simulink model "pr733_DUC_modulation"  (R2018b)
settings: Solver=VariableStepAuto  StartTime=0.0  StopTime=8192/fs  RelTol=1e-3
PreLoadFcn:
  | fs=1e8;
  | pr731_DUC_setup;
  | fc=40e6;
undefined symbols (not defined in the file or in its folder): CFIR, CIC, designMultirateFIR, RRC
libraries: dspmlti4 x6, commrandsrc3 x1, commdigbbndpm3 x1
settings Model: Creator=Григорий Фокин  LastModifiedBy=Григорий Фокин
settings DataIOCC: SaveFormat=Array  SaveOutput=off  SignalLogging=off  SaveTime=off
settings DebuggingCC: AlgebraicLoopMsg=error
settings HardwareCC: ProdBitPerPointer=32  ProdBitPerSizeT=32  ProdBitPerPtrDiffT=32  ProdLargestAtomicFloat=None  ProdIntDivRoundTo=Undefined  ProdEndianess=Unspecified  ProdWordSize=32  ProdHWDeviceType=ASIC/FPGA->ASIC/FPGA  TargetBitPerPointer=64  TargetBitPerSizeT=64  TargetBitPerPtrDiffT=64  TargetLongLongMode=on  TargetIntDivRoundTo=Zero  TargetEndianess=LittleEndian  TargetWordSize=64  TargetHWDeviceType=Custom Processor->MATLAB Host Computer  ProdEqTarget=off

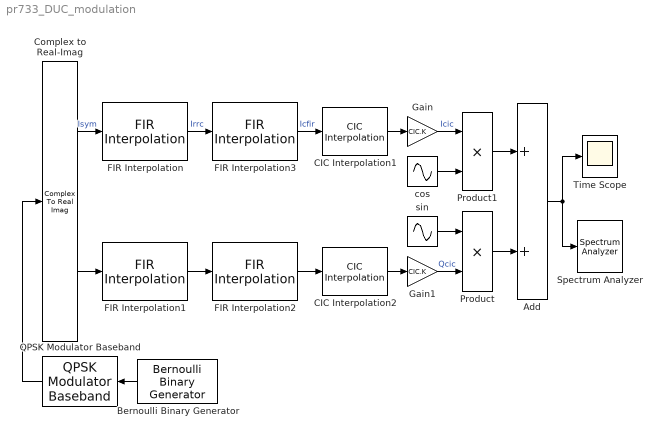
== system pr733_DUC_modulation ==
  Add : Sum
  Bernoulli Binary Generator : commrandsrc3/Bernoulli Binary Generator  ProbabilityOfZero=0.5  SeedSource=Auto  Seed=0  SampleTime=(0.5*CIC.R*RRC.Lfactor*CFIR.Lfactor)/fs  SamplesPerFrame=2  OutputDataType=boolean  SimulateUsing=Interpreted execution
  CIC Interpolation1 : dspmlti4/CIC Interpolation  filtFrom=Multirate object in workspace  filtobj=hCIC  ftype=Interpolator  R=2  M=1  N=2  filterInternals=Full precision  BPS=[16 16 16 16]  FLPS=0  outputWordLength=32  outputFracLength=0  launchFVT=off  framing=Allow multirate processing  OutputFrames=off
      settings: SourceProductName=DSP System Toolbox  SourceProductBaseCode=DS
  CIC Interpolation2 : dspmlti4/CIC Interpolation  filtFrom=Multirate object in workspace  filtobj=hCIC  ftype=Interpolator  R=2  M=1  N=2  filterInternals=Full precision  BPS=[16 16 16 16]  FLPS=0  outputWordLength=32  outputFracLength=0  launchFVT=off  framing=Allow multirate processing  OutputFrames=off
      settings: SourceProductName=DSP System Toolbox  SourceProductBaseCode=DS
  Complex to Real-Imag : ComplexToRealImag
  FIR Interpolation : dspmlti4/FIR Interpolation  FilterSource=Filter object  h=designMultirateFIR(3,1)  L=3  FilterObject=hRRC  framing=Enforce single-rate processing  outputBufInitCond=0  roundingMode=Floor  overflowMode=off  firstCoeffDataTypeStr=Inherit: Same word length as input  firstCoeffMin=[]  firstCoeffMax=[]  firstCoeffLastDataTypeStr=Inherit: Same word length as input  outputDataTypeStr=Inherit: Same as accumulator  outputMin=[]  outputMax=[]  outputLastDataTypeStr=Inherit: Same as accumulator
      settings: SourceProductName=DSP System Toolbox
  FIR Interpolation1 : dspmlti4/FIR Interpolation  FilterSource=Filter object  h=designMultirateFIR(3,1)  L=3  FilterObject=hRRC  framing=Enforce single-rate processing  outputBufInitCond=0  roundingMode=Floor  overflowMode=off  firstCoeffDataTypeStr=Inherit: Same word length as input  firstCoeffMin=[]  firstCoeffMax=[]  firstCoeffLastDataTypeStr=Inherit: Same word length as input  outputDataTypeStr=Inherit: Same as accumulator  outputMin=[]  outputMax=[]  outputLastDataTypeStr=Inherit: Same as accumulator
      settings: SourceProductName=DSP System Toolbox
  FIR Interpolation2 : dspmlti4/FIR Interpolation  FilterSource=Filter object  h=designMultirateFIR(3,1)  L=3  FilterObject=hCFIR  framing=Enforce single-rate processing  outputBufInitCond=0  roundingMode=Floor  overflowMode=off  firstCoeffDataTypeStr=Inherit: Same word length as input  firstCoeffMin=[]  firstCoeffMax=[]  firstCoeffLastDataTypeStr=Inherit: Same word length as input  outputDataTypeStr=Inherit: Same as accumulator  outputMin=[]  outputMax=[]  outputLastDataTypeStr=Inherit: Same as accumulator
      settings: SourceProductName=DSP System Toolbox
  FIR Interpolation3 : dspmlti4/FIR Interpolation  FilterSource=Filter object  h=designMultirateFIR(3,1)  L=3  FilterObject=hCFIR  framing=Enforce single-rate processing  outputBufInitCond=0  roundingMode=Floor  overflowMode=off  firstCoeffDataTypeStr=Inherit: Same word length as input  firstCoeffMin=[]  firstCoeffMax=[]  firstCoeffLastDataTypeStr=Inherit: Same word length as input  outputDataTypeStr=Inherit: Same as accumulator  outputMin=[]  outputMax=[]  outputLastDataTypeStr=Inherit: Same as accumulator
      settings: SourceProductName=DSP System Toolbox
  Gain : Gain  Gain=CIC.K  OutMin=-1  OutMax=1  OutDataTypeStr=fixdt(1,16)
  Gain1 : Gain  Gain=CIC.K  OutMin=-1  OutMax=1  OutDataTypeStr=fixdt(1,16)
  Product : Product
  Product1 : Product
  QPSK Modulator Baseband : commdigbbndpm3/QPSK Modulator Baseband  InType=Bit  Enc=Gray  Ph=pi/4  outDtype=Fixed-point  outWordLen=16  outUDDataType=sfix(16)  outFracLenMode=Best precision  outFracLen=15  outDataTypeStr=fixdt(1,16)  outLastDataTypeStr=fixdt(1,16)
  Spectrum Analyzer : SpectrumAnalyzer
  Time Scope : Scope
  cos : Sin  Frequency=fc*2*pi  Phase=pi/2  SampleTime=1/fs
  sin : Sin  Frequency=fc*2*pi  SampleTime=1/fs
  wires:
  Bernoulli Binary Generator/1 -> QPSK Modulator Baseband/1
  QPSK Modulator Baseband/1 -> Complex to Real-Imag/1
  Complex to Real-Imag/1 -> FIR Interpolation/1  "Isym"
  Complex to Real-Imag/2 -> FIR Interpolation1/1
  FIR Interpolation1/1 -> FIR Interpolation2/1
  FIR Interpolation/1 -> FIR Interpolation3/1  "Irrc"
  FIR Interpolation3/1 -> CIC Interpolation1/1  "Icfir"
  FIR Interpolation2/1 -> CIC Interpolation2/1
  CIC Interpolation2/1 -> Gain1/1
  CIC Interpolation1/1 -> Gain/1
  Gain1/1 -> Product/2  "Qcic"
  Gain/1 -> Product1/1  "Icic"
  cos/1 -> Product1/2
  sin/1 -> Product/1
  Product/1 -> Add/2
  Product1/1 -> Add/1
  Add/1 -> Time Scope/1, Spectrum Analyzer/1
